simulink model "game_monitor"  (R2017a)
settings: Solver=FixedStepAuto  StartTime=0.0  StopTime=inf  FixedStep=0.2  RelTol=1e-3
libraries: robotlib x3
settings Model: Creator=Aurelio.Bermudez  LastModifiedBy=Aurelio.Bermudez

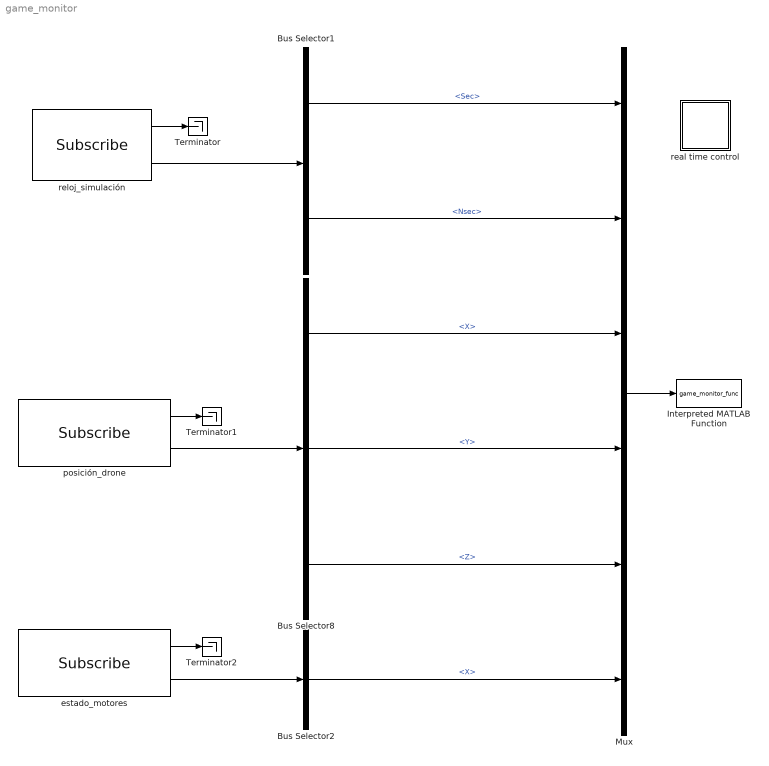
== system game_monitor ==
  Bus Selector1 : BusSelector  DialogController=Simulink.DDGSource_BusSelector  OutputSignals=Clock_.Sec,Clock_.Nsec
  Bus Selector2 : BusSelector  DialogController=Simulink.DDGSource_BusSelector  OutputSignals=Position.X
  Bus Selector8 : BusSelector  DialogController=Simulink.DDGSource_BusSelector  OutputSignals=Pose.Position.X,Pose.Position.Y,Pose.Position.Z
  Interpreted MATLAB Function : MATLABFcn  MATLABFcn=game_monitor_func  OutputDimensions=0
  Mux : Mux  Inputs=6
  Terminator : Terminator
  Terminator1 : Terminator
  Terminator2 : Terminator
  estado_motores : robotlib/Subscribe  SourceLibraryInfo=This block requires Robotics System Toolbox  topicSource=Select from ROS network  topic=/quadcopter/bus_command  messageType=geometry_msgs/Pose  sampleTime=-1  messageQueueLength=1
      settings: SourceProductBaseCode=RO
  posición_drone : robotlib/Subscribe  SourceLibraryInfo=This block requires Robotics System Toolbox  topicSource=Select from ROS network  topic=/quadcopter/odometry  messageType=gazebo_msgs/ModelState  sampleTime=-1  messageQueueLength=1
      settings: SourceProductBaseCode=RO
  real time control : Subsystem
      mask Display: disp('realtime\ncontrol')
  reloj_simulación : robotlib/Subscribe  SourceLibraryInfo=This block requires Robotics System Toolbox  topicSource=Select from ROS network  topic=/clock  messageType=rosgraph_msgs/Clock  sampleTime=-1  messageQueueLength=1
      settings: SourceProductBaseCode=RO
  wires:
  reloj_simulación/2 -> Bus Selector1/1
  posición_drone/2 -> Bus Selector8/1
  Mux/1 -> Interpreted MATLAB Function/1
  estado_motores/2 -> Bus Selector2/1
  Bus Selector8/3 -> Mux/5  "<Z>"
  Bus Selector8/2 -> Mux/4  "<Y>"
  Bus Selector8/1 -> Mux/3  "<X>"
  Bus Selector1/1 -> Mux/1  "<Sec>"
  Bus Selector1/2 -> Mux/2  "<Nsec>"
  reloj_simulación/1 -> Terminator/1
  posición_drone/1 -> Terminator1/1
  estado_motores/1 -> Terminator2/1
  Bus Selector2/1 -> Mux/6  "<X>"

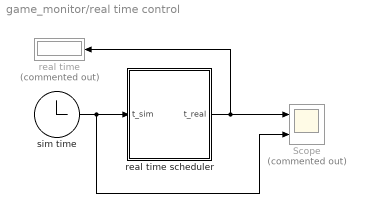
== system game_monitor/real time control ==
  Scope : Scope  Commented=on  NumInputPorts=2
  real time : Display  Commented=on
      settings: Format=bank
  real time scheduler : MATLAB Function  TreatAsAtomicUnit=on
  sim time : Clock
  wires:
  real time scheduler/1(t_real) -> real time/1, Scope/1
  sim time/1 -> real time scheduler/1(t_sim), Scope/2

== matlab function game_monitor/real time control/real time scheduler ==
  data: t_sim input; t_real output
function t_real = fcn(t_sim)
%#codegen

coder.extrinsic('tic');
coder.extrinsic('toc');

persistent t0;
if isempty(t0)
    t0 = tic;
    t_real = 0;
end

t_real = toc(t0);

t_dif = t_sim - t_real;
if t_dif > 0
%    disp(t_dif)
    pause(t_dif);
end

t_real = toc(t0);
%disp(t_real)
